simulink subsystem "eqorientation"  (R2023a)
settings: Solver=VariableStepAuto  StartTime=0.0  StopTime=10.0  RelTol=1e-3
undefined symbols (not defined in the file or in its folder): I
libraries: matrix_library x1
settings Model: Creator=ccubertou  LastModifiedBy=raphb

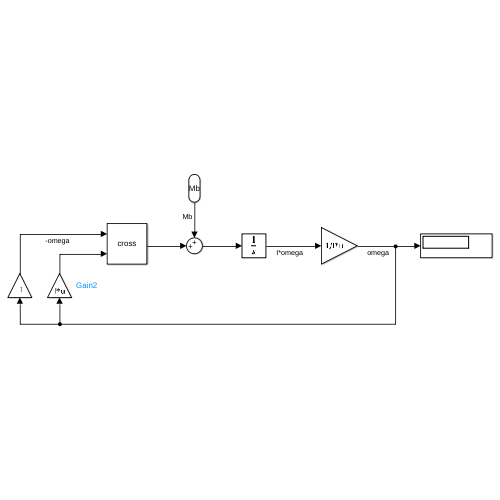
[thumbnail: Simulink's stored preview of the top-level diagram]
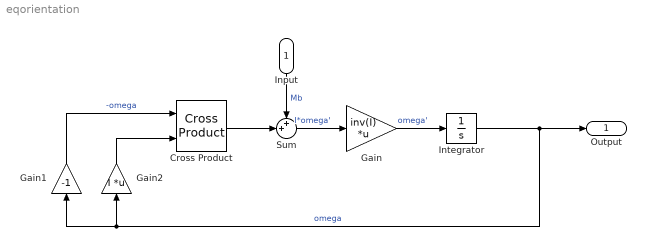
== system eqorientation ==
  Input : Inport
  Cross Product : matrix_library/Cross Product
  Gain : Gain  Gain=inv(I)  Multiplication=Matrix(K*u)
  Gain1 : Gain  Gain=-1
  Gain2 : Gain  Gain=I  Multiplication=Matrix(K*u)
  Integrator : Integrator
  Sum : Sum  Inputs=++|
  Output : Outport
  wires:
  Sum/1 -> Gain/1  "I*omega'"
  Gain/1 -> Integrator/1  "omega'"
  Gain1/1 -> Cross Product/1  "-omega"
  Gain2/1 -> Cross Product/2
  Input/1 -> Sum/1  "Mb"
  Cross Product/1 -> Sum/2
  Integrator/1 -> Gain1/1, Gain2/1, Output/1  "omega"
